simulink model "pfc"  (R2022b)
settings: Solver=VariableStepAuto  StartTime=0.0  StopTime=10.0  RelTol=1e-3
values from neighbouring files (symbols this model uses):
  Ts = 1e-7    (= 1e-07)    [pfc_init.m]
libraries: spsDiodeLib x4, peripheral_utilities x4, spsSeriesRLCBranchLib x3, spsControlledVoltageSourceLib x1, spsGroundLib x1, spspowerguiLib x1
settings Model: Creator=javnson  LastModifiedBy=javnson

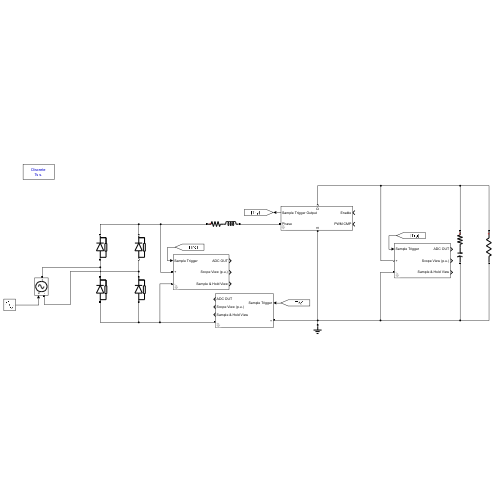
[thumbnail: Simulink's stored preview of the top-level diagram]
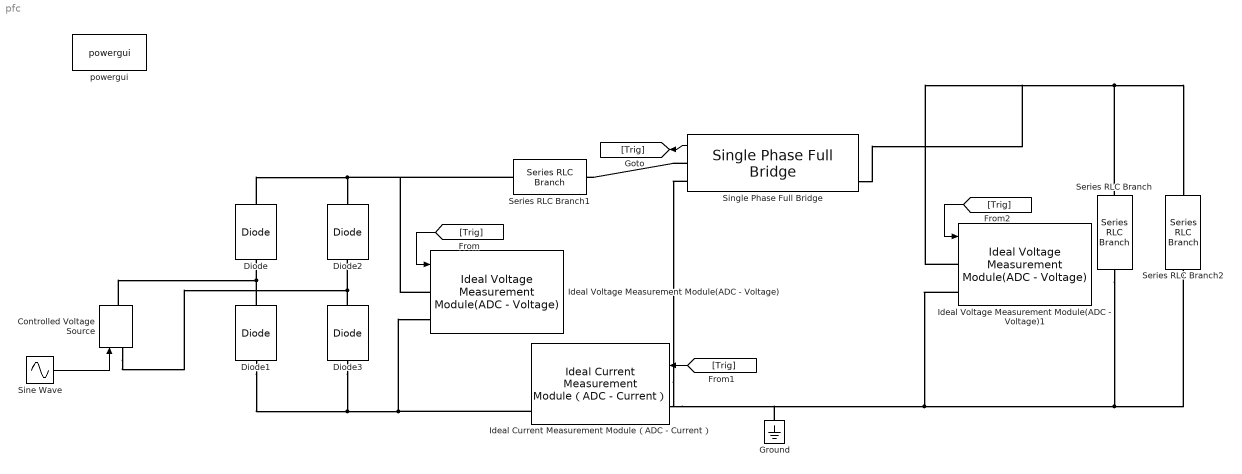
== system pfc ==
  Controlled Voltage Source : spsControlledVoltageSourceLib/Controlled Voltage Source  Initialize=on  Source_Type=AC  Amplitude=0  Phase=0  Frequency=0  Measurements=None
  Diode{,1..3} (4 alike) : spsDiodeLib/Diode  Ron=0.001  Lon=0  Vf=0.8  IC=0  UseSnubber=0  Rs=500  Cs=250e-9  Measurements=off
  Ground : spsGroundLib/Ground  LConnTagsString=a
  Ideal Current Measurement Module（ADC - Current） : peripheral_utilities/Ideal Current Measurement Module（ADC - Current）  ADC_GAIN=1  ADC_BIT=16  ADC_REFERENCE=20.0  ADC_BIAS=10  ADC_INIT=0
      settings: SourceProductName=GMP Utilities Library
  Ideal Voltage Measurement Module(ADC - Voltage) : peripheral_utilities/Ideal Voltage Measurement Module(ADC - Voltage)  ADC_GAIN=1/10  ADC_BIT=16  ADC_REFERENCE=3  ADC_BIAS=0  ADC_INIT=0
      settings: SourceProductName=GMP Utilities Library
  Ideal Voltage Measurement Module(ADC - Voltage)1 : peripheral_utilities/Ideal Voltage Measurement Module(ADC - Voltage)  ADC_GAIN=1/10  ADC_BIT=16  ADC_REFERENCE=3  ADC_BIAS=0  ADC_INIT=0
      settings: SourceProductName=GMP Utilities Library
  Series RLC Branch : spsSeriesRLCBranchLib/Series RLC Branch  LConnTagsString=__new0  RConnTagsString=__new0  BranchType=RC  Resistance=1  Inductance=1e-3  SetiL0=off  InitialCurrent=0  Capacitance=1e-6  Setx0=off  InitialVoltage=0  Measurements=None
  Series RLC Branch1 : spsSeriesRLCBranchLib/Series RLC Branch  LConnTagsString=__new0  RConnTagsString=__new0  BranchType=RL  Resistance=1  Inductance=1e-3  SetiL0=off  InitialCurrent=0  Capacitance=1e-6  Setx0=off  InitialVoltage=0  Measurements=None
  Series RLC Branch2 : spsSeriesRLCBranchLib/Series RLC Branch  LConnTagsString=__new0  RConnTagsString=__new0  BranchType=R  Resistance=1  Inductance=1e-3  SetiL0=off  InitialCurrent=0  Capacitance=1e-6  Setx0=off  InitialVoltage=0  Measurements=None
  Sine Wave : Sin  SampleTime=0
  Single Phase Full Bridge : peripheral_utilities/Single Phase Full Bridge  fswitch=10e3  CMP_MAX=10000  Deadband_Upper=100  Deadband_Lower=100  Deadband_us=1  phase_shift=0  R_mosfet_on=0.1  Lon=0  Rd=0.01  Vf=0.3  Rs=1e5  Cs=inf
      settings: SourceProductName=GMP Utilities Library
  powergui : spspowerguiLib/powergui  Priority=1  SimulationMode=Discrete  SampleTime=Ts  frequency=60  Iterations=50  frequencyindice=60  Pbase=100e6  ErrMax=1e-4  UnitsV=kV  UnitsW=MW  buscounter=0  FunctionMessages=off  echomessages=off  EnableUseOfTLC=off  CurrentSourceSwitches=off  DisableSnubberDevices=off  DisableRonSwitches=off  DisableVfSwitches=off  DisplayEquations=off  AutomaticDiscreteSolvers=off  SolverType=Tustin/Backward Euler (TBE)  Interpol=off  ExternalGateDelay=off  methode=off  Ts=100  x0status=blocks  SPID=on  SwTol=0  HookPort=off  NonlinearTolerance=1e-4  nMaxIteration=100  ContinueOnMaxIteration=off  RestoreLinks=warning  ResistiveCurrentMeasurement=off  Frange=[0:2:500]  Ylog=off  Xlog=on  ShowGrid=off  save=off  variable=ZData  structure=0  ZoomFFT=off  StartTime=0.0  cycles=1  DisplayStyle=1  fundamental=60  FreqAxis=off  MaxFrequency=1000  frequencyindicesteady=1  RmsSteady=1  display=off
  wires:
  Sine Wave/1 -> Controlled Voltage Source/1
  Single Phase Full Bridge/1 -> [Trig]
  [Trig] -> Ideal Voltage Measurement Module(ADC - Voltage)/1
  [Trig] -> Ideal Current Measurement Module（ADC - Current）/1
  [Trig] -> Ideal Voltage Measurement Module(ADC - Voltage)1/1
  connections:
  Diode1/RConn1 -- Controlled Voltage Source/RConn1 -- Diode/LConn1
  Diode3/RConn1 -- Controlled Voltage Source/LConn1 -- Diode2/LConn1
  Series RLC Branch/RConn1 -- Ideal Voltage Measurement Module(ADC - Voltage)1/LConn2 -- Single Phase Full Bridge/RConn2 -- Ideal Current Measurement Module（ADC - Current）/LConn1 -- Ground/LConn1 -- Series RLC Branch2/RConn1
  Diode/RConn1 -- Ideal Voltage Measurement Module(ADC - Voltage)/LConn1 -- Series RLC Branch1/LConn1 -- Diode2/RConn1
  Series RLC Branch/LConn1 -- Ideal Voltage Measurement Module(ADC - Voltage)1/LConn1 -- Single Phase Full Bridge/LConn1 -- Series RLC Branch2/LConn1
  Single Phase Full Bridge/RConn1 -- Series RLC Branch1/RConn1
  Diode3/LConn1 -- Diode1/LConn1 -- Ideal Voltage Measurement Module(ADC - Voltage)/LConn2 -- Ideal Current Measurement Module（ADC - Current）/RConn1
